simulink library "gmp_sil_core_pack_src"  (R2022b)
settings: Solver=VariableStepAuto  StartTime=0.0  StopTime=10.0  RelTol=1e-3
libraries: gmp_sil_core_pack x3
settings Model: Creator=javnson  LastModifiedBy=javnson

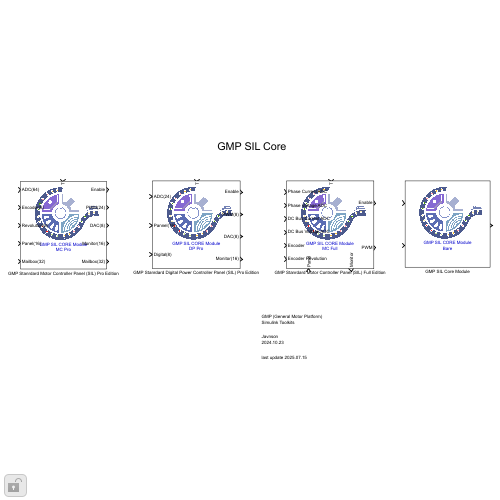
[thumbnail: Simulink's stored preview of the top-level diagram]
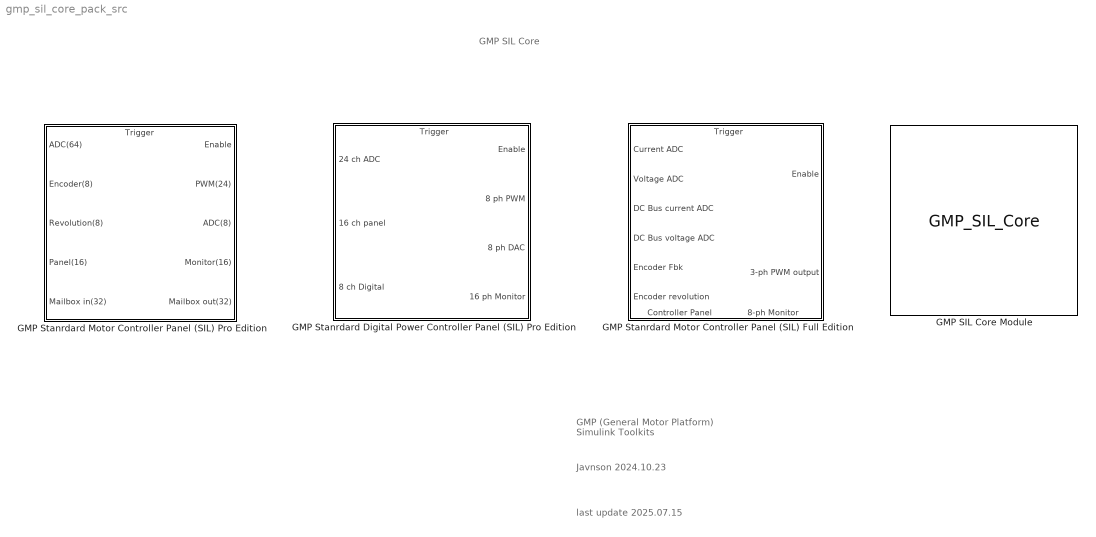
== system gmp_sil_core_pack_src ==
  note: last update 2025.07.15
  note: GMP SIL Core
  note: Javnson
      | 2024.10.23
  note: GMP (General Motor Platform)
      | Simulink Toolkits
  GMP SIL Core Module : S-Function  FunctionName=GMP_SIL_Core  Parameters=NumberUnpackedPorts, UnpackedDataTypes, UnpackedDataSizes, NumberPackedPorts, PackedDataTypes, PackedDataSizes, Alignment, HostAddr, TargetPort  SFunctionDeploymentMode=off  EnableBusSupport=off  mask(GMP CTL SIL Core){MaskPackedDataTypes={'double','double'}, MaskPackedDataSizes={[1],[1]}, MaskUnpackedDataTypes={'double'}, MaskUnpackedDataSizes={[1]}, MaskAlignment=1, MaskHostAddr='127.0.0.1', MaskMsgTxPort=12300, MaskMsgRxPort=12301, MaskCmdTxPort=12302, MaskCmdRxPort=12303}
      mask help:
      | This is the GMP (General Motor Platform) CTL (Control Template Library) SIL (Software In Loop) Core Model.
      | User should fill the following communication settings.
      mask init:
      | % MDL invoke parameters
      | % NumberUnpackedPorts, UnpackedDataTypes, UnpackedDataSizes, 
      | % NumberPackedPorts, PackedDataTypes, PackedDataSizes, 
      | % Alignment,
      | % HostAddr, TargetPort
      | 
      | % source: MaskUnpackedDataTypes, MaskUnpackedDataSizes
      | % source: MaskPackedDataTypes, MaskUnpackedDataSizes
      | % source: MaskAlignment
      | [NumberUnpackedPorts, UnpackedDataTypes, UnpackedDataSizes, ...
      |      NumberPackedPorts, PackedDataTypes, PackedDataSizes, ...
      |      Alignment] = mdl_gmp_simulink_core( ...
      |      MaskUnpackedDataTypes, MaskUnpackedDataSizes, ...
      |      MaskPackedDataTypes, MaskPackedDataSizes,...
      |      MaskAlignment);
      | 
      | % source: MaskHostAddr
      | % source: MaskMsgTxPort, MaskMsgRxPort
      | % source: MaskCmdTxPort, MaskCmdRxPort
      | [HostAddr, TargetPort] = mdl_gmp_simulink_connection(MaskHostAddr, ...
      | 	MaskMsgTxPort, MaskMsgRxPort, ... 
      | 	MaskCmdTxPort, MaskCmdRxPort);
      mask TypeOptions MaskAlignment: 1 | 2 | 4 | 8
      mask DialogControl ParameterGroupVar Prompt: Parameters:
      mask DialogControl Container5 Prompt: Message
      mask DialogControl Control3 Prompt: Data (sent) types (cell array):(pack)
      mask DialogControl Control7 Prompt: Data (send) port dimisions (cell array) (pack), disabled
      mask DialogControl Control5 Prompt: Data (received) types (cell array):(unpack)
      mask DialogControl Control6 Prompt: Data (received) port dimisions (cell array)(unpacked)
      mask DialogControl Control4 Prompt: Byte Alignment:
      mask DialogControl Container6 Prompt: Connection
      mask DialogControl Control8 Prompt: Target Host:
      mask DialogControl Control9 Prompt: MSG Transmit Port:
      mask DialogControl Control10 Prompt: MSG Receive Port:
      mask DialogControl Container7 Prompt: Command Ports
      mask DialogControl Control11 Prompt: CMD Transmit Port:
      mask DialogControl Control12 Prompt: CMD Receive Port:
      mask Display:
      | image(append(fileparts(which('gmp_simulink_utilities.slx')),'\icon\GMP_Core.png'));
      | 
      | color('blue');
      | disp('\n\n\n\n\n\n\n\nGMP SIL CORE Module\nBare');
      | 
      | 
      | color('Black');
  GMP Stanrdard Digital Power Controller Panel (SIL) Pro Edition : Subsystem  mask(GMP SIL Core for single Motor Controller (full edition)){}
      mask help: This is GMP Motor Simulator port.
      settings: PortSchema="{\"entries\":[{\"content\":{\"sides\":[{\"content\":{\"connectorIds\":[\"In1\",\"In2\",\"In3\"]},\"type\":\"ConnectorPlacement.EquallySpacedRectSide\",\"uuid\":\"45c67bc9-9540-469a-a4ac-1e12eb9acca3\"},{\"content\":{\"connectorIds\":[\"Out1\",\"Out2\",\"Out3\",\"Out4\"],\"side\":\"RIGHT\"},\"type\":\"ConnectorPlacement.EquallySpacedRectSide\",\"uuid\":\"a17116b4-0460-48ab-8ada-a785da6c5e29\"},{\"content\":{\"connectorIds\":[\"In4\"],\"side\":\"TOP\"},\"type\":\"ConnectorPlacement.EquallySpacedRectSide\",\"uuid\":\"15623697-512e-4e4d-ab51-f53c2346fadb\"},{\"content\":{\"side\":\"BOTTOM\"},\"type\":\"ConnectorPlacement.EquallySpacedRectSide\",\"uuid\":\"47f7968c-22c1-4f3d-97d9-242e9dbf8d30\"}]},\"type\":\"ConnectorPlacement.EquallySpacedConnector\",\"uuid\":\"f369880c-e675-4c1f-982e-a4befb03f503\"}],\"packageUris\":[\"http://schema.mathworks.com/mf0/Connector/R2020b\"],\"version\":\"1.0\"}"
      mask DialogControl ParameterGroupVar Prompt: 参数
      mask Display:
      | image(append(fileparts(which('gmp_simulink_utilities.slx')),'\icon\GMP_Core.png'));
      | color('blue');
      | %text(0.3,0.3,'GMP SIL CORE Module','horizontalAlignment','left','verticalAlignment','bottom');
      | disp('\n\n\n\n\n\n\n\nGMP SIL CORE Module\nDP Pro');
      | %text(0,0,'y=a*x^2+b','horizontalAlignment','middle', 'verticalAlignment','bottom');
      | 
      | 
      | module_pos = get_param(gcb, 'Position');
      | width = module_pos(3) - module_pos(1);
      | %rectangle('Position',[module_pos(1),module_pos(2),module_pos(3),module_pos(4)],'FaceColor','r');
      | 
      | color('Black');
      | 
      | port_label('output', 1, 'Enable');
      | port_label('output', 2, 'PWM(8)');
      | port_label('output', 3, 'DAC(8)');
      | port_label('output', 4, 'Monitor(16)');
      | 
      | port_label('input', 1, 'ADC(24)');
      | port_label('input', 2, 'Pannel(16)');
      | port_label('input', 3, 'Digital(8)');
      | port_label('input', 4, 'T');
  GMP Stanrdard Motor Controller Panel (SIL) Full Edition : Subsystem  mask(GMP SIL Core for single Motor Controller (full edition)){}
      mask help: This is GMP Motor Simulator port.
      settings: PortSchema="{\"entries\":[{\"content\":{\"sides\":[{\"content\":{\"connectorIds\":[\"In1\",\"In2\",\"In3\",\"In4\",\"In5\",\"In6\"]},\"type\":\"ConnectorPlacement.EquallySpacedRectSide\",\"uuid\":\"45c67bc9-9540-469a-a4ac-1e12eb9acca3\"},{\"content\":{\"connectorIds\":[\"Out1\",\"Out2\"],\"side\":\"RIGHT\"},\"type\":\"ConnectorPlacement.EquallySpacedRectSide\",\"uuid\":\"a17116b4-0460-48ab-8ada-a785da6c5e29\"},{\"content\":{\"connectorIds\":[\"In7\"],\"side\":\"TOP\"},\"type\":\"ConnectorPlacement.EquallySpacedRectSide\",\"uuid\":\"15623697-512e-4e4d-ab51-f53c2346fadb\"},{\"content\":{\"connectorIds\":[\"In8\",\"Out3\"],\"side\":\"BOTTOM\"},\"type\":\"ConnectorPlacement.EquallySpacedRectSide\",\"uuid\":\"47f7968c-22c1-4f3d-97d9-242e9dbf8d30\"}]},\"type\":\"ConnectorPlacement.EquallySpacedConnector\",\"uuid\":\"f369880c-e675-4c1f-982e-a4befb03f503\"}],\"packageUris\":[\"http://schema.mathworks.com/mf0/Connector/R2020b\"],\"version\":\"1.0\"}"
      mask DialogControl ParameterGroupVar Prompt: 参数
      mask Display:
      | image(append(fileparts(which('gmp_simulink_utilities.slx')),'\icon\GMP_Core.png'));
      | color('blue');
      | %text(0.3,0.3,'GMP SIL CORE Module','horizontalAlignment','left','verticalAlignment','bottom');
      | disp('\n\n\n\n\n\n\n\nGMP SIL CORE Module\nMC Full');
      | %text(0,0,'y=a*x^2+b','horizontalAlignment','middle', 'verticalAlignment','bottom');
      | 
      | 
      | module_pos = get_param(gcb, 'Position');
      | width = module_pos(3) - module_pos(1);
      | %rectangle('Position',[module_pos(1),module_pos(2),module_pos(3),module_pos(4)],'FaceColor','r');
      | 
      | color('Black');
      | 
      | port_label('output', 1, 'Enable');
      | port_label('output', 2, 'PWM');
      | port_label('output', 3, 'Monitor');
      | 
      | port_label('input', 1, 'Phase Current ADC');
      | port_label('input', 2, 'Phase Voltage ADC');
      | port_label('input', 3, 'DC Bus Current ADC');
      | port_label('input', 4, 'DC Bus Voltage ADC');
      | port_label('input', 5, 'Encoder');
      | port_label('input', 6, 'Encoder Revolution');
      | port_label('input', 7, 'T');
      | port_label('input', 8, 'Panel');
  GMP Stanrdard Motor Controller Panel (SIL) Pro Edition : Subsystem  mask(GMP SIL Core for single Motor Controller (Pro edition)){}
      mask help:
      | This is GMP Motor Simulator port.
      | This module is for multi motor simulation.
      settings: PortSchema="{\"entries\":[{\"content\":{\"sides\":[{\"content\":{\"connectorIds\":[\"In1\",\"In2\",\"In3\",\"In4\",\"In5\"]},\"type\":\"ConnectorPlacement.EquallySpacedRectSide\",\"uuid\":\"bbb38fc4-c00d-4f5b-8f26-db6bc7dcef4b\"},{\"content\":{\"connectorIds\":[\"Out1\",\"Out2\",\"Out3\",\"Out4\",\"Out5\"],\"side\":\"RIGHT\"},\"type\":\"ConnectorPlacement.EquallySpacedRectSide\",\"uuid\":\"8c76eb91-b69b-4328-81e2-2047f2677c46\"},{\"content\":{\"connectorIds\":[\"In6\"],\"side\":\"TOP\"},\"type\":\"ConnectorPlacement.EquallySpacedRectSide\",\"uuid\":\"10c40072-39ff-4b1a-b98b-8537349958a4\"}]},\"type\":\"ConnectorPlacement.EquallySpacedConnector\",\"uuid\":\"17ad35a3-8880-4c96-99ea-a2d74561424d\"}],\"packageUris\":[\"http://schema.mathworks.com/mf0/Connector/R2020b\"],\"version\":\"1.0\"}"
      mask DialogControl ParameterGroupVar Prompt: 参数
      mask Display:
      | image(append(fileparts(which('gmp_simulink_utilities.slx')),'\icon\GMP_Core.png'));
      | color('blue');
      | %text(0.3,0.3,'GMP SIL CORE Module','horizontalAlignment','left','verticalAlignment','bottom');
      | disp(['\n\n\n\n\n\n\n\nGMP SIL CORE Module\nMC Pro']);
      | %text(0,0,'y=a*x^2+b','horizontalAlignment','middle', 'verticalAlignment','bottom');
      | 
      | 
      | module_pos = get_param(gcb, 'Position');
      | width = module_pos(3) - module_pos(1);
      | %rectangle('Position',[module_pos(1),module_pos(2),module_pos(3),module_pos(4)],'FaceColor','r');
      | 
      | color('Black');
      | 
      | port_label('output', 1, 'Enable');
      | port_label('output', 2, 'PWM(24)');
      | port_label('output', 3, 'DAC(8)');
      | port_label('output', 4, 'Monitor(16)');
      | port_label('output', 5, 'Mailbox(32)');
      | 
      | port_label('input', 1, 'ADC(64)');
      | port_label('input', 2, 'Encoder(8)');
      | port_label('input', 3, 'Revolution(8)');
      | port_label('input', 4, 'Panel(16)');
      | port_label('input', 5, 'Mailbox(32)');
      | port_label('input', 6, 'T');

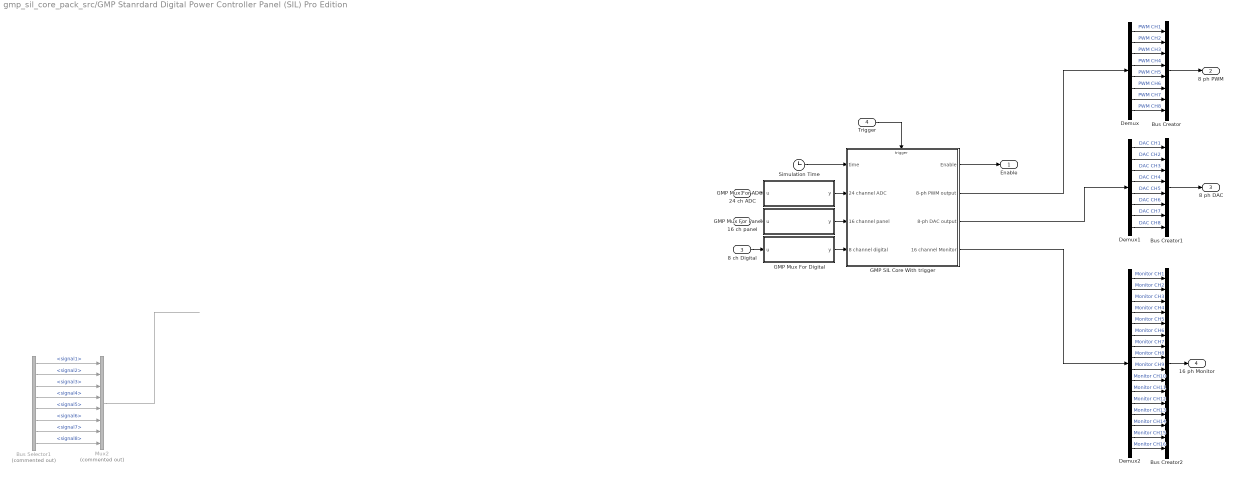
== system gmp_sil_core_pack_src/GMP Stanrdard Digital Power Controller Panel (SIL) Pro Edition ==
  24 ch ADC : Inport
  16 ch panel : Inport  Port=2
  8 ch Digital : Inport  Port=3
  Trigger : Inport  Port=4
  Bus Creator : BusCreator  Inputs=8
  Bus Creator1 : BusCreator  Inputs=8
  Bus Creator2 : BusCreator  Inputs=16
  Bus Selector1 : BusSelector  Commented=on  OutputSignals=signal1,signal2,signal3,signal4,signal5,signal6,signal7,signal8
  Demux : Demux  Outputs=8
  Demux1 : Demux  Outputs=8
  Demux2 : Demux  Outputs=16
  GMP Mux For ADC : MATLAB Function  TreatAsAtomicUnit=on
  GMP Mux For Digital : MATLAB Function  TreatAsAtomicUnit=on
  GMP Mux For Panel : MATLAB Function  TreatAsAtomicUnit=on
  GMP SIL Core With trigger : Subsystem
  Mux2 : Mux  Commented=on  Inputs=8
  Simulation Time : Clock
  Enable : Outport
  8 ph PWM : Outport  Port=2
  8 ph DAC : Outport  Port=3
  16 ph Monitor : Outport  Port=4
  wires:
  Simulation Time/1 -> GMP SIL Core With trigger/1(time)
  GMP SIL Core With trigger/1(Enable) -> Enable/1
  Trigger/1 -> GMP SIL Core With trigger/Trigger
  Demux/1 -> Bus Creator/1  "PWM CH1"
  Demux/2 -> Bus Creator/2  "PWM CH2"
  Demux/3 -> Bus Creator/3  "PWM CH3"
  Demux/4 -> Bus Creator/4  "PWM CH4"
  Demux/5 -> Bus Creator/5  "PWM CH5"
  Demux/6 -> Bus Creator/6  "PWM CH6"
  Demux/7 -> Bus Creator/7  "PWM CH7"
  Demux/8 -> Bus Creator/8  "PWM CH8"
  Demux1/8 -> Bus Creator1/8  "DAC CH8"
  Demux1/7 -> Bus Creator1/7  "DAC CH7"
  Demux1/6 -> Bus Creator1/6  "DAC CH6"
  Demux1/5 -> Bus Creator1/5  "DAC CH5"
  Demux1/4 -> Bus Creator1/4  "DAC CH4"
  Demux1/3 -> Bus Creator1/3  "DAC CH3"
  Demux1/2 -> Bus Creator1/2  "DAC CH2"
  Demux1/1 -> Bus Creator1/1  "DAC CH1"
  Demux2/1 -> Bus Creator2/1  "Monitor CH1"
  Demux2/2 -> Bus Creator2/2  "Monitor CH2"
  Demux2/3 -> Bus Creator2/3  "Monitor CH3"
  Demux2/4 -> Bus Creator2/4  "Monitor CH4"
  Demux2/5 -> Bus Creator2/5  "Monitor CH5"
  Demux2/6 -> Bus Creator2/6  "Monitor CH6"
  Demux2/7 -> Bus Creator2/7  "Monitor CH7"
  Demux2/8 -> Bus Creator2/8  "Monitor CH8"
  Demux2/9 -> Bus Creator2/9  "Monitor CH9"
  Demux2/10 -> Bus Creator2/10  "Monitor CH10"
  Demux2/11 -> Bus Creator2/11  "Monitor CH11"
  Demux2/12 -> Bus Creator2/12  "Monitor CH12"
  Demux2/13 -> Bus Creator2/13  "Monitor CH13"
  Demux2/14 -> Bus Creator2/14  "Monitor CH14"
  Demux2/15 -> Bus Creator2/15  "Monitor CH15"
  Demux2/16 -> Bus Creator2/16  "Monitor CH16"
  Bus Creator2/1 -> 16 ph Monitor/1
  GMP SIL Core With trigger/4(16 channel Monitor) -> Demux2/1
  Bus Creator1/1 -> 8 ph DAC/1
  GMP SIL Core With trigger/3(8-ph DAC output) -> Demux1/1
  Bus Creator/1 -> 8 ph PWM/1
  GMP SIL Core With trigger/2(8-ph PWM output) -> Demux/1
  Mux2/1 -> ?
  ? -> Bus Selector1/1
  Bus Selector1/4 -> Mux2/4  "<signal4>"
  Bus Selector1/1 -> Mux2/1  "<signal1>"
  Bus Selector1/7 -> Mux2/7  "<signal7>"
  Bus Selector1/6 -> Mux2/6  "<signal6>"
  Bus Selector1/3 -> Mux2/3  "<signal3>"
  Bus Selector1/8 -> Mux2/8  "<signal8>"
  Bus Selector1/5 -> Mux2/5  "<signal5>"
  Bus Selector1/2 -> Mux2/2  "<signal2>"
  GMP Mux For Digital/1(y) -> GMP SIL Core With trigger/4(8 channel digital)
  8 ch Digital/1 -> GMP Mux For Digital/1(u)
  16 ch panel/1 -> GMP Mux For Panel/1(u)
  GMP Mux For Panel/1(y) -> GMP SIL Core With trigger/3(16 channel panel)
  24 ch ADC/1 -> GMP Mux For ADC/1(u)
  GMP Mux For ADC/1(y) -> GMP SIL Core With trigger/2(24 channel ADC)

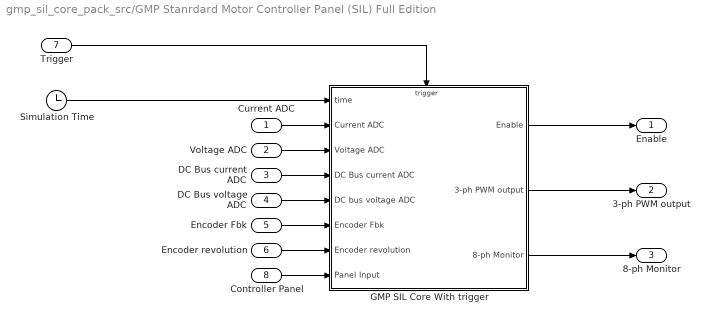
== system gmp_sil_core_pack_src/GMP Stanrdard Motor Controller Panel (SIL) Full Edition ==
  Current ADC : Inport
  Voltage ADC : Inport  Port=2
  DC Bus current ADC : Inport  Port=3
  DC Bus voltage ADC : Inport  Port=4
  Encoder Fbk : Inport  Port=5
  Encoder revolution : Inport  Port=6
  Trigger : Inport  Port=7
  Controller Panel : Inport  Port=8
  GMP SIL Core With trigger : Subsystem
  Simulation Time : Clock
  Enable : Outport
  3-ph PWM output : Outport  Port=2
  8-ph Monitor : Outport  Port=3
  wires:
  Encoder Fbk/1 -> GMP SIL Core With trigger/6(Encoder Fbk)
  Encoder revolution/1 -> GMP SIL Core With trigger/7(Encoder revolution)
  GMP SIL Core With trigger/2(3-ph PWM output) -> 3-ph PWM output/1
  Simulation Time/1 -> GMP SIL Core With trigger/1(time)
  GMP SIL Core With trigger/1(Enable) -> Enable/1
  Voltage ADC/1 -> GMP SIL Core With trigger/3(Voltage ADC)
  Current ADC/1 -> GMP SIL Core With trigger/2(Current ADC)
  GMP SIL Core With trigger/3(8-ph Monitor) -> 8-ph Monitor/1
  DC Bus current ADC/1 -> GMP SIL Core With trigger/4(DC Bus current ADC)
  Trigger/1 -> GMP SIL Core With trigger/Trigger
  DC Bus voltage ADC/1 -> GMP SIL Core With trigger/5(DC bus voltage ADC)
  Controller Panel/1 -> GMP SIL Core With trigger/8(Panel Input)

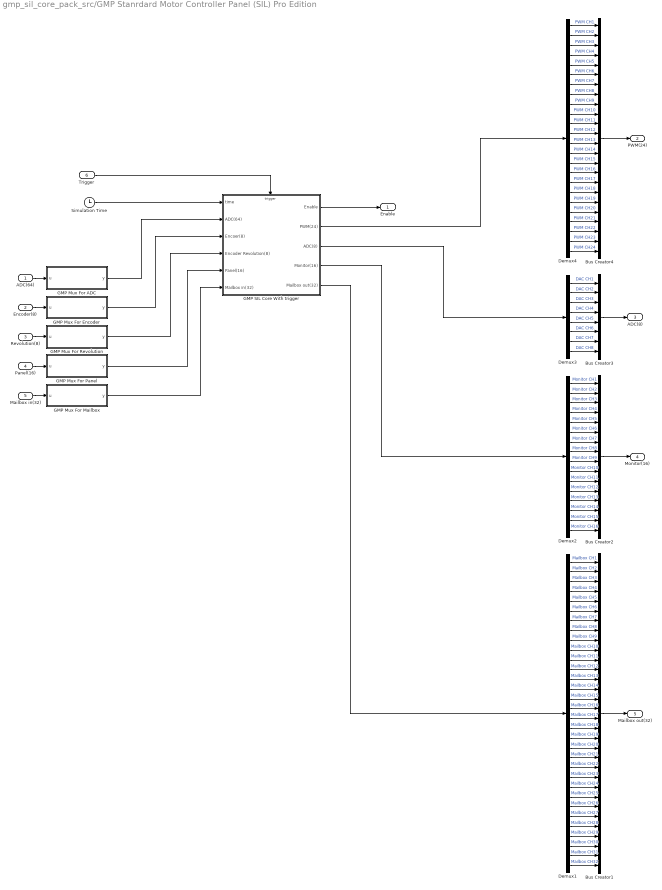
== system gmp_sil_core_pack_src/GMP Stanrdard Motor Controller Panel (SIL) Pro Edition ==
  ADC(64) : Inport
  Encoder(8) : Inport  Port=2
  Revolution(8) : Inport  Port=3
  Panel(16) : Inport  Port=4
  Mailbox in(32) : Inport  Port=5
  Trigger : Inport  Port=6
  Bus Creator1 : BusCreator  Inputs=32
  Bus Creator2 : BusCreator  Inputs=16
  Bus Creator3 : BusCreator  Inputs=8
  Bus Creator4 : BusCreator  Inputs=24
  Demux1 : Demux  Outputs=32
  Demux2 : Demux  Outputs=16
  Demux3 : Demux  Outputs=8
  Demux4 : Demux  Outputs=24
  GMP Mux For ADC : MATLAB Function  TreatAsAtomicUnit=on
  GMP Mux For Encoder : MATLAB Function  TreatAsAtomicUnit=on
  GMP Mux For Mailbox : MATLAB Function  TreatAsAtomicUnit=on
  GMP Mux For Panel : MATLAB Function  TreatAsAtomicUnit=on
  GMP Mux For Revolution : MATLAB Function  TreatAsAtomicUnit=on
  GMP SIL Core With trigger : Subsystem
  Simulation Time : Clock
  Enable : Outport
  PWM(24) : Outport  Port=2
  ADC(8) : Outport  Port=3
  Monitor(16) : Outport  Port=4
  Mailbox out(32) : Outport  Port=5
  wires:
  GMP SIL Core With trigger/1(Enable) -> Enable/1
  Trigger/1 -> GMP SIL Core With trigger/Trigger
  Simulation Time/1 -> GMP SIL Core With trigger/1(time)
  Mailbox in(32)/1 -> GMP Mux For Mailbox/1(u)
  Panel(16)/1 -> GMP Mux For Panel/1(u)
  Encoder(8)/1 -> GMP Mux For Encoder/1(u)
  Revolution(8)/1 -> GMP Mux For Revolution/1(u)
  ADC(64)/1 -> GMP Mux For ADC/1(u)
  GMP Mux For ADC/1(y) -> GMP SIL Core With trigger/2(ADC(64))
  GMP Mux For Encoder/1(y) -> GMP SIL Core With trigger/3(Encoer(8))
  GMP Mux For Revolution/1(y) -> GMP SIL Core With trigger/4(Encoder Revolution(8))
  GMP Mux For Panel/1(y) -> GMP SIL Core With trigger/5(Panel(16))
  GMP Mux For Mailbox/1(y) -> GMP SIL Core With trigger/6(Mailbox in(32))
  Demux2/10 -> Bus Creator2/10  "Monitor CH10"
  Demux2/5 -> Bus Creator2/5  "Monitor CH5"
  Demux2/7 -> Bus Creator2/7  "Monitor CH7"
  Demux2/8 -> Bus Creator2/8  "Monitor CH8"
  Demux2/9 -> Bus Creator2/9  "Monitor CH9"
  Demux2/13 -> Bus Creator2/13  "Monitor CH13"
  Demux2/12 -> Bus Creator2/12  "Monitor CH12"
  Demux2/11 -> Bus Creator2/11  "Monitor CH11"
  GMP SIL Core With trigger/4(Monitor(16)) -> Demux2/1
  Demux2/16 -> Bus Creator2/16  "Monitor CH16"
  Demux2/3 -> Bus Creator2/3  "Monitor CH3"
  Demux2/4 -> Bus Creator2/4  "Monitor CH4"
  Demux2/6 -> Bus Creator2/6  "Monitor CH6"
  Demux2/2 -> Bus Creator2/2  "Monitor CH2"
  Demux2/15 -> Bus Creator2/15  "Monitor CH15"
  Demux2/14 -> Bus Creator2/14  "Monitor CH14"
  Demux2/1 -> Bus Creator2/1  "Monitor CH1"
  Bus Creator2/1 -> Monitor(16)/1
  Demux1/14 -> Bus Creator1/14  "Mailbox CH14"
  Demux1/1 -> Bus Creator1/1  "Mailbox CH1"
  Demux1/4 -> Bus Creator1/4  "Mailbox CH4"
  GMP SIL Core With trigger/5(Mailbox out(32)) -> Demux1/1
  Demux1/6 -> Bus Creator1/6  "Mailbox CH6"
  Demux1/11 -> Bus Creator1/11  "Mailbox CH11"
  Demux1/3 -> Bus Creator1/3  "Mailbox CH3"
  Demux1/16 -> Bus Creator1/16  "Mailbox CH16"
  Demux1/2 -> Bus Creator1/2  "Mailbox CH2"
  Demux1/13 -> Bus Creator1/13  "Mailbox CH13"
  Demux1/5 -> Bus Creator1/5  "Mailbox CH5"
  Demux1/7 -> Bus Creator1/7  "Mailbox CH7"
  Demux1/10 -> Bus Creator1/10  "Mailbox CH10"
  Demux1/9 -> Bus Creator1/9  "Mailbox CH9"
  Demux1/12 -> Bus Creator1/12  "Mailbox CH12"
  Demux1/15 -> Bus Creator1/15  "Mailbox CH15"
  Bus Creator1/1 -> Mailbox out(32)/1
  Demux1/8 -> Bus Creator1/8  "Mailbox CH8"
  Demux1/17 -> Bus Creator1/17  "Mailbox CH17"
  Demux1/18 -> Bus Creator1/18  "Mailbox CH18"
  Demux1/19 -> Bus Creator1/19  "Mailbox CH19"
  Demux1/20 -> Bus Creator1/20  "Mailbox CH20"
  Demux1/21 -> Bus Creator1/21  "Mailbox CH21"
  Demux1/22 -> Bus Creator1/22  "Mailbox CH22"
  Demux1/23 -> Bus Creator1/23  "Mailbox CH23"
  Demux1/24 -> Bus Creator1/24  "Mailbox CH24"
  Demux1/25 -> Bus Creator1/25  "Mailbox CH25"
  Demux1/26 -> Bus Creator1/26  "Mailbox CH26"
  Demux1/27 -> Bus Creator1/27  "Mailbox CH27"
  Demux1/28 -> Bus Creator1/28  "Mailbox CH28"
  Demux1/29 -> Bus Creator1/29  "Mailbox CH29"
  Demux1/30 -> Bus Creator1/30  "Mailbox CH30"
  Demux1/31 -> Bus Creator1/31  "Mailbox CH31"
  Demux1/32 -> Bus Creator1/32  "Mailbox CH32"
  Demux3/2 -> Bus Creator3/2  "DAC CH2"
  Demux3/5 -> Bus Creator3/5  "DAC CH5"
  Demux3/3 -> Bus Creator3/3  "DAC CH3"
  Demux3/7 -> Bus Creator3/7  "DAC CH7"
  Demux3/8 -> Bus Creator3/8  "DAC CH8"
  Demux3/4 -> Bus Creator3/4  "DAC CH4"
  Demux3/1 -> Bus Creator3/1  "DAC CH1"
  Bus Creator3/1 -> ADC(8)/1
  Demux3/6 -> Bus Creator3/6  "DAC CH6"
  GMP SIL Core With trigger/3(ADC(8)) -> Demux3/1
  Demux4/8 -> Bus Creator4/8  "PWM CH8"
  Demux4/15 -> Bus Creator4/15  "PWM CH15"
  Demux4/12 -> Bus Creator4/12  "PWM CH12"
  Demux4/9 -> Bus Creator4/9  "PWM CH9"
  Demux4/7 -> Bus Creator4/7  "PWM CH7"
  Demux4/5 -> Bus Creator4/5  "PWM CH5"
  Demux4/10 -> Bus Creator4/10  "PWM CH10"
  Demux4/13 -> Bus Creator4/13  "PWM CH13"
  Demux4/2 -> Bus Creator4/2  "PWM CH2"
  Demux4/16 -> Bus Creator4/16  "PWM CH16"
  Demux4/6 -> Bus Creator4/6  "PWM CH6"
  GMP SIL Core With trigger/2(PWM(24)) -> Demux4/1
  Demux4/11 -> Bus Creator4/11  "PWM CH11"
  Demux4/14 -> Bus Creator4/14  "PWM CH14"
  Demux4/24 -> Bus Creator4/24  "PWM CH24"
  Demux4/19 -> Bus Creator4/19  "PWM CH19"
  Demux4/23 -> Bus Creator4/23  "PWM CH23"
  Demux4/1 -> Bus Creator4/1  "PWM CH1"
  Bus Creator4/1 -> PWM(24)/1
  Demux4/20 -> Bus Creator4/20  "PWM CH20"
  Demux4/21 -> Bus Creator4/21  "PWM CH21"
  Demux4/22 -> Bus Creator4/22  "PWM CH22"
  Demux4/3 -> Bus Creator4/3  "PWM CH3"
  Demux4/17 -> Bus Creator4/17  "PWM CH17"
  Demux4/18 -> Bus Creator4/18  "PWM CH18"
  Demux4/4 -> Bus Creator4/4  "PWM CH4"

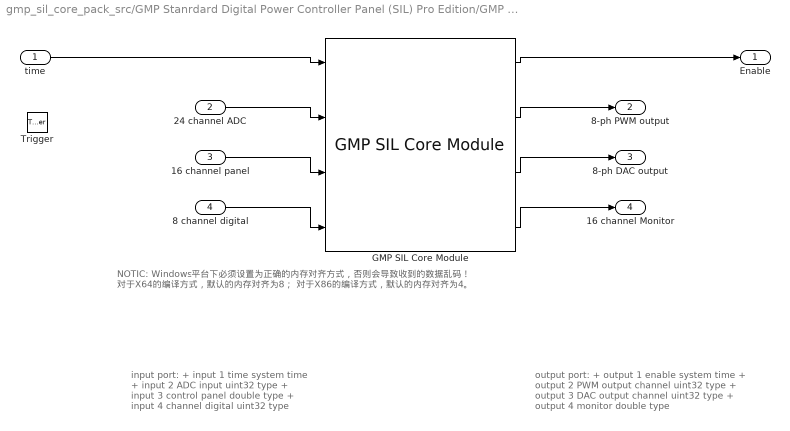
== system gmp_sil_core_pack_src/GMP Stanrdard Digital Power Controller Panel (SIL) Pro Edition/GMP SIL Core With trigger ==
  note: input port:
      | + input 1 time system time
      | + input 2 ADC input uint32 type
      | + input 3 control panel double type
      | + input 4 channel digital uint32 type
  note: NOTIC:
      | Windows平台下必须设置为正确的内存对齐方式，否则会导致收到的数据乱码！
      | 对于X64的编译方式，默认的内存对齐为8；
      | 对于X86的编译方式，默认的内存对齐为4。
  note: output port:
      | + output 1 enable system time
      | + output 2 PWM output channel uint32 type
      | + output 3 DAC output channel uint32 type
      | + output 4 monitor double type
  time : Inport
  24 channel ADC : Inport  Port=2
  16 channel panel : Inport  Port=3
  8 channel digital : Inport  Port=4
  Trigger : TriggerPort  VariantControl=(inherit)  PortDimensions=1
  GMP SIL Core Module : gmp_sil_core_pack/GMP SIL Core Module  MaskPackedDataTypes={'double', 'uint32', 'double', 'int32'}  MaskPackedDataSizes={[1],[24],[16],[8]}  MaskUnpackedDataTypes={'double', 'uint32', 'uint32', 'double'}  MaskUnpackedDataSizes={[1],[8],[8],[16]}  MaskAlignment=1  MaskHostAddr='127.0.0.1'  MaskMsgTxPort=12500  MaskMsgRxPort=12501  MaskCmdTxPort=12502  MaskCmdRxPort=12503
      settings: SourceProductName=GMP SIL Core Utilities
  Enable : Outport
  8-ph PWM output : Outport  Port=2
  8-ph DAC output : Outport  Port=3
  16 channel Monitor : Outport  Port=4
  wires:
  24 channel ADC/1 -> GMP SIL Core Module/2
  16 channel panel/1 -> GMP SIL Core Module/3
  time/1 -> GMP SIL Core Module/1
  GMP SIL Core Module/3 -> 8-ph DAC output/1
  GMP SIL Core Module/2 -> 8-ph PWM output/1
  GMP SIL Core Module/1 -> Enable/1
  8 channel digital/1 -> GMP SIL Core Module/4
  GMP SIL Core Module/4 -> 16 channel Monitor/1

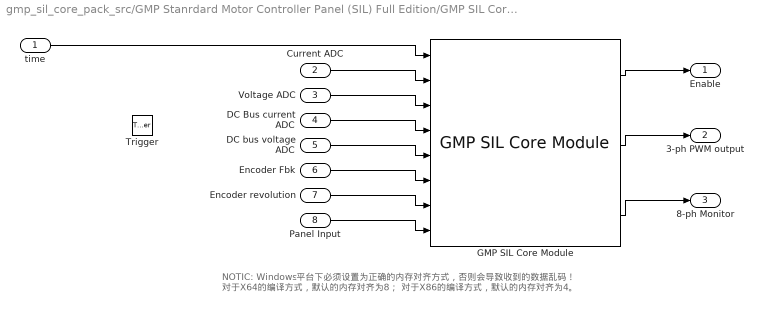
== system gmp_sil_core_pack_src/GMP Stanrdard Motor Controller Panel (SIL) Full Edition/GMP SIL Core With trigger ==
  note: NOTIC:
      | Windows平台下必须设置为正确的内存对齐方式，否则会导致收到的数据乱码！
      | 对于X64的编译方式，默认的内存对齐为8；
      | 对于X86的编译方式，默认的内存对齐为4。
  time : Inport
  Current ADC : Inport  Port=2
  Voltage ADC : Inport  Port=3
  DC Bus current ADC : Inport  Port=4
  DC bus voltage ADC : Inport  Port=5
  Encoder Fbk : Inport  Port=6
  Encoder revolution : Inport  Port=7
  Panel Input : Inport  Port=8
  Trigger : TriggerPort  VariantControl=(inherit)  PortDimensions=1
  GMP SIL Core Module : gmp_sil_core_pack/GMP SIL Core Module  MaskPackedDataTypes={'double','uint32','uint32','uint32','uint32', 'uint32', 'int32', 'double'}  MaskPackedDataSizes={[1],[3],[3],[1],[1], [1], [1], [4]}  MaskUnpackedDataTypes={'double', 'uint32','double'}  MaskUnpackedDataSizes={[1],[3],[8]}  MaskAlignment=1  MaskHostAddr='127.0.0.1'  MaskMsgTxPort=12300  MaskMsgRxPort=12301  MaskCmdTxPort=12302  MaskCmdRxPort=12303
      settings: SourceProductName=GMP SIL Core Utilities
  Enable : Outport
  3-ph PWM output : Outport  Port=2
  8-ph Monitor : Outport  Port=3
  wires:
  Current ADC/1 -> GMP SIL Core Module/2
  Voltage ADC/1 -> GMP SIL Core Module/3
  DC Bus current ADC/1 -> GMP SIL Core Module/4
  time/1 -> GMP SIL Core Module/1
  GMP SIL Core Module/3 -> 8-ph Monitor/1
  GMP SIL Core Module/2 -> 3-ph PWM output/1
  GMP SIL Core Module/1 -> Enable/1
  Encoder Fbk/1 -> GMP SIL Core Module/6
  Encoder revolution/1 -> GMP SIL Core Module/7
  DC bus voltage ADC/1 -> GMP SIL Core Module/5
  Panel Input/1 -> GMP SIL Core Module/8

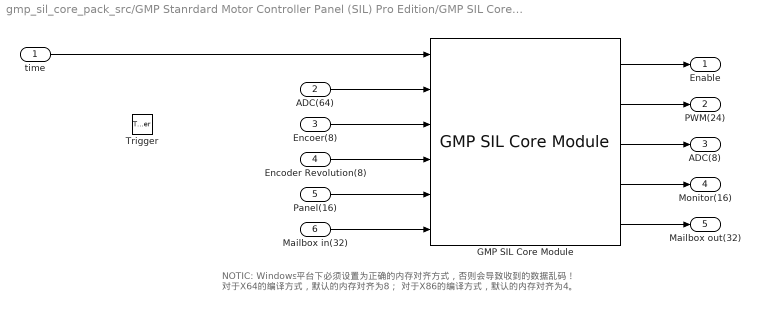
== system gmp_sil_core_pack_src/GMP Stanrdard Motor Controller Panel (SIL) Pro Edition/GMP SIL Core With trigger ==
  note: NOTIC:
      | Windows平台下必须设置为正确的内存对齐方式，否则会导致收到的数据乱码！
      | 对于X64的编译方式，默认的内存对齐为8；
      | 对于X86的编译方式，默认的内存对齐为4。
  time : Inport
  ADC(64) : Inport  Port=2
  Encoer(8) : Inport  Port=3
  Encoder Revolution(8) : Inport  Port=4
  Panel(16) : Inport  Port=5
  Mailbox in(32) : Inport  Port=6
  Trigger : TriggerPort  VariantControl=(inherit)  PortDimensions=1
  GMP SIL Core Module : gmp_sil_core_pack/GMP SIL Core Module  MaskPackedDataTypes={'double','uint32','uint32', 'int32', 'double', 'int32'}  MaskPackedDataSizes={[1],[64],[8],[8],[16], [32]}  MaskUnpackedDataTypes={'double', 'uint32','uint32','double','int32'}  MaskUnpackedDataSizes={[1],[24],[8],[16],[32]}  MaskAlignment=1  MaskHostAddr='127.0.0.1'  MaskMsgTxPort=12300  MaskMsgRxPort=12301  MaskCmdTxPort=12302  MaskCmdRxPort=12303
      settings: SourceProductName=GMP SIL Core Utilities
  Enable : Outport
  PWM(24) : Outport  Port=2
  ADC(8) : Outport  Port=3
  Monitor(16) : Outport  Port=4
  Mailbox out(32) : Outport  Port=5
  wires:
  Panel(16)/1 -> GMP SIL Core Module/5
  Mailbox in(32)/1 -> GMP SIL Core Module/6
  GMP SIL Core Module/1 -> Enable/1
  GMP SIL Core Module/2 -> PWM(24)/1
  GMP SIL Core Module/3 -> ADC(8)/1
  time/1 -> GMP SIL Core Module/1
  Encoder Revolution(8)/1 -> GMP SIL Core Module/4
  Encoer(8)/1 -> GMP SIL Core Module/3
  ADC(64)/1 -> GMP SIL Core Module/2
  GMP SIL Core Module/4 -> Monitor(16)/1
  GMP SIL Core Module/5 -> Mailbox out(32)/1

== matlab function gmp_sil_core_pack_src/GMP Stanrdard Digital Power Controller Panel (SIL) Pro Edition/GMP Mux For Panel ==
  data: u input; y output
function y = gmp_mux_util(u)

size = 16;

size_u = length(u);

%typename_of_u = class(u(1));
typename_of_u = 'double';

z = zeros(size- size_u, 1, typename_of_u);

y = [u;z];

== matlab function gmp_sil_core_pack_src/GMP Stanrdard Digital Power Controller Panel (SIL) Pro Edition/GMP Mux For ADC ==
  data: u input; y output
function y = gmp_mux_util(u)

size = 24;

size_u = length(u);

%typename_of_u = class(u(1));
typename_of_u = 'uint32';

z = zeros(size- size_u, 1, typename_of_u);

y = [u;z];

== matlab function gmp_sil_core_pack_src/GMP Stanrdard Motor Controller Panel (SIL) Pro Edition/GMP Mux For Mailbox ==
  data: u input; y output
function y = gmp_mux_util(u)

size = 32;

size_u = length(u);

%typename_of_u = class(u(1));
typename_of_u = 'int32';

z = zeros(size- size_u, 1, typename_of_u);

y = [u;z];

== matlab function gmp_sil_core_pack_src/GMP Stanrdard Motor Controller Panel (SIL) Pro Edition/GMP Mux For Panel ==
  data: u input; y output
function y = gmp_mux_util(u)

size = 16;

size_u = length(u);

%typename_of_u = class(u(1));
typename_of_u = 'double';

z = zeros(size- size_u, 1, typename_of_u);

y = [u;z];

== matlab function gmp_sil_core_pack_src/GMP Stanrdard Motor Controller Panel (SIL) Pro Edition/GMP Mux For Revolution ==
  data: u input; y output
function y = gmp_mux_util(u)

size = 8;

size_u = length(u);

%typename_of_u = class(u(1));
typename_of_u = 'int32';

z = zeros(size- size_u, 1, typename_of_u);

y = [u;z];

== matlab function gmp_sil_core_pack_src/GMP Stanrdard Motor Controller Panel (SIL) Pro Edition/GMP Mux For Encoder ==
  data: u input; y output
function y = gmp_mux_util(u)

size = 8;

size_u = length(u);

%typename_of_u = class(u(1));
typename_of_u = 'uint32';

z = zeros(size- size_u, 1, typename_of_u);

y = [u;z];

== matlab function gmp_sil_core_pack_src/GMP Stanrdard Motor Controller Panel (SIL) Pro Edition/GMP Mux For ADC ==
  data: u input; y output
function y = gmp_mux_util(u)

size = 64;

size_u = length(u);

%typename_of_u = class(u(1));
typename_of_u = 'uint32';

z = zeros(size- size_u, 1, typename_of_u);

y = [u;z];

== matlab function gmp_sil_core_pack_src/GMP Stanrdard Digital Power Controller Panel (SIL) Pro Edition/GMP Mux For Digital ==
  data: u input; y output
function y = gmp_mux_util(u)

size = 8;

size_u = length(u);

%typename_of_u = class(u(1));
typename_of_u = 'int32';

z = zeros(size- size_u, 1, typename_of_u);

y = [u;z];
